simulink library "f14actuator"  (Simulink 6.0)
settings: Solver=ode45  SolverMode=SingleTasking  StartTime=0.0  StopTime=10.0  RelTol=1e-3
values from neighbouring files (symbols this model uses):
  Ta = 0.05    [autopilot_data.mat]    (also in f14dat.m; f14def.m)
libraries: f14actuator x1
settings Model: Creator=The MathWorks Inc.  LastModifiedBy=batserve  ExtModeAutoUpdateStatusClock=off
settings OptimizationCC: BooleanDataType=off
settings DebuggingCC: CheckExecutionContextPreStartOutputMsg=on  CheckExecutionContextRuntimeOutputMsg=on  SolverPrmCheckMsg=none
settings HardwareCC: TargetUnknown=on

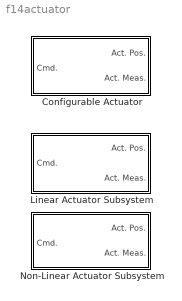
== system f14actuator ==
  Configurable Actuator : Subsystem  BlockChoice=Linear Actuator Subsystem  PropExecContextAcrossSSBoundary=on
      settings: TemplateBlock=self  MemberBlocks=Linear Actuator Subsystem,Non-Linear Actuator Subsystem
  Linear Actuator Subsystem : Subsystem  PropExecContextAcrossSSBoundary=on
      mask Display: text(0.5,0.5,'[Linear]','horizontalAlignment','center');
  Non-Linear Actuator Subsystem : Subsystem  PropExecContextAcrossSSBoundary=on
      mask Display: text(0.5,0.5,'[Non-Linear]','horizontalAlignment','center')

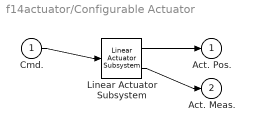
== system f14actuator/Configurable Actuator ==
  Cmd. : Inport  Port=1  LatchInput=off
  Linear Actuator Subsystem : f14actuator/Linear Actuator Subsystem
  Act. Pos. : Outport
  Act. Meas. : Outport  Port=2
  wires:
  Cmd./1 -> Linear Actuator Subsystem/1
  Linear Actuator Subsystem/1 -> Act. Pos./1
  Linear Actuator Subsystem/2 -> Act. Meas./1

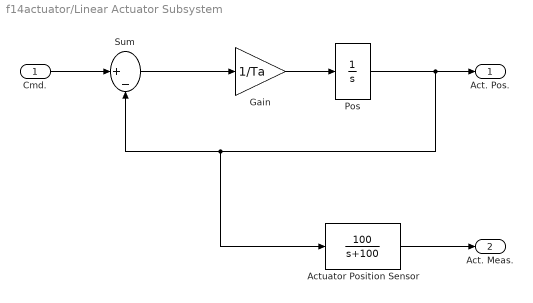
== system f14actuator/Linear Actuator Subsystem ==
  Cmd. : Inport  Port=1  LatchInput=off
  Actuator Position Sensor : TransferFcn  Numerator=[100]  Denominator=[1 100]
  Gain : Gain  Gain=1/Ta  SaturateOnIntegerOverflow=on
  Pos : Integrator  UpperSaturationLimit=pi*45/180  LowerSaturationLimit=-pi*45/180
  Sum : Sum  Inputs=|+-  SaturateOnIntegerOverflow=on  InputSameDT=on
  Act. Pos. : Outport  InitialOutput=0
  Act. Meas. : Outport  Port=2  InitialOutput=0
  wires:
  Actuator Position Sensor/1 -> Act. Meas./1
  Cmd./1 -> Sum/1
  Pos/1 -> Act. Pos./1, Actuator Position Sensor/1, Sum/2
  Gain/1 -> Pos/1
  Sum/1 -> Gain/1

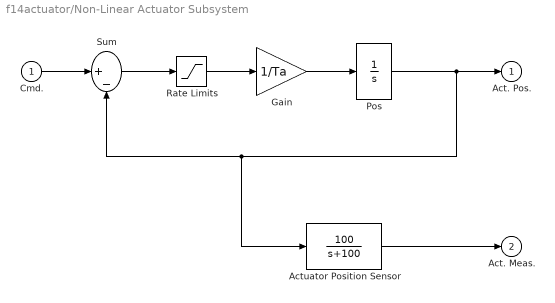
== system f14actuator/Non-Linear Actuator Subsystem ==
  Cmd. : Inport  Port=1  LatchInput=off
  Actuator Position Sensor : TransferFcn  Numerator=[100]  Denominator=[1 100]
  Gain : Gain  Gain=1/Ta  SaturateOnIntegerOverflow=on
  Pos : Integrator  LimitOutput=on  UpperSaturationLimit=pi*45/180  LowerSaturationLimit=-pi*45/180
  Rate Limits : Saturate
  Sum : Sum  Inputs=|+-  SaturateOnIntegerOverflow=on  InputSameDT=on
  Act. Pos. : Outport  InitialOutput=0
  Act. Meas. : Outport  Port=2  InitialOutput=0
  wires:
  Actuator Position Sensor/1 -> Act. Meas./1
  Pos/1 -> Act. Pos./1, Actuator Position Sensor/1, Sum/2
  Cmd./1 -> Sum/1
  Sum/1 -> Rate Limits/1
  Gain/1 -> Pos/1
  Rate Limits/1 -> Gain/1
